simulink model "linCartPendulum"  (R2026a)
settings: Solver=VariableStepAuto
values from neighbouring files (symbols this model uses):
  A = inv([1 0 0 0; 0 1 0 0; 0 0 M+m -m*l; 0 0 -m*l J+m*l^2])*[0 0 1 0; 0 0 0 1; 0 0 -c 0; 0 m*g*l 0 -gamma]    [setupModelParameters.m]
  B = inv([1 0 0 0; 0 1 0 0; 0 0 M+m -m*l; 0 0 -m*l J+m*l^2])*[0; 0; 1; 0]    [setupModelParameters.m]
  C = eye(4, 4)    [setupModelParameters.m]
  D = zeros(4, 1)    [setupModelParameters.m]
  K = place(A, B, desired_poles)    [setupModelParameters.m]
  kr = -inv(Cp*inv(A-B*K)*B)    [setupModelParameters.m]
  xinit = [0;0.8;0;0]    [setupModelParameters.m]
settings Model: Creator=jamess  LastModifiedBy=socks

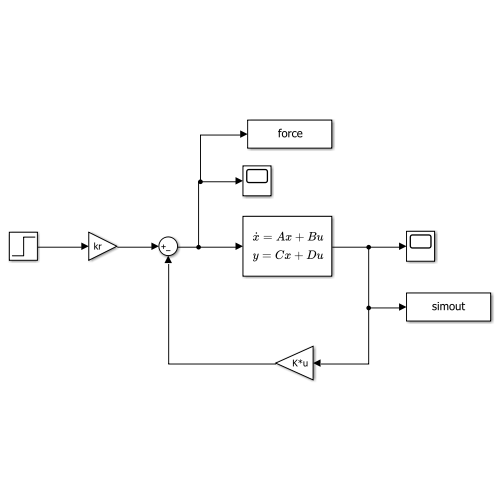
[thumbnail: Simulink's stored preview of the top-level diagram]
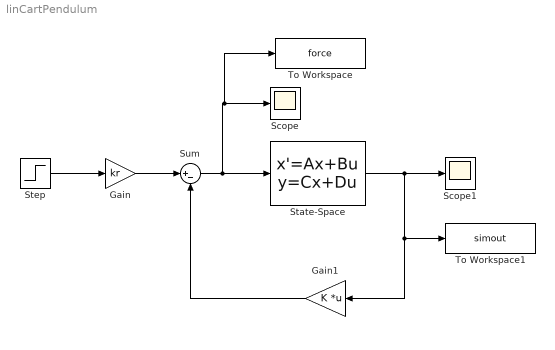
== system linCartPendulum ==
  Gain : Gain  Gain=kr
  Gain1 : Gain  Gain=K  Multiplication=Matrix(K*u)
  Scope : Scope
      settings: ActiveDisplayYMinimum=-12.83176609782633  ActiveDisplayYMaximum=16.157484840558993
  Scope1 : Scope
      settings: ActiveDisplayYMinimum=-0.89519191641624885  ActiveDisplayYMaximum=1.6194573503473486
  State-Space : StateSpace  A=A  B=B  C=C  D=D  InitialCondition=xinit
  Step : Step  Time=0  FinalValue=stepFinal  SampleTime=0
  Sum : Sum  Inputs=|+-
  To Workspace : ToWorkspace  VariableName=force  SaveFormat=Timeseries  SampleTime=-1
  To Workspace1 : ToWorkspace  VariableName=simout  SaveFormat=Timeseries  SampleTime=-1
  wires:
  State-Space/1 -> To Workspace1/1, Gain1/1, Scope1/1
  Sum/1 -> To Workspace/1, Scope/1, State-Space/1
  Gain/1 -> Sum/1
  Step/1 -> Gain/1
  Gain1/1 -> Sum/2
